simulink model "px42LoopCtr20210902"  (R2022a)
settings: Solver=FixedStepDiscrete  StartTime=0.0  StopTime=inf  FixedStep=0.005  RelTol=1e-3  EnableMultiTasking=on
InitFcn:
  | I_x = 0.00478;
  | I_y = 0.00502;
  | I_z = 0.00736;
  | m=1;
  | L=0.11667;
undefined symbols (not defined in the file): dev, DiscIntNeverNeededParam, Main, pwm_output0
libraries: simulink x30, px4lib x3, px4uORBlib x2, sharedtransform x1
(part 1 of 3)
settings Model: SimulationMode=external  ExtModeTrigDuration=10  Creator=The MathWorks, Inc.  LastModifiedBy=001
settings SolverCC: AlgebraicLoopSolver=TrustRegion  PositivePriorityOrder=on  AutoInsertRateTranBlk=on
settings DataIOCC: LimitDataPoints=on  MaxDataPoints=10000
settings OptimizationCC: BlockReduction=off  EnhancedBackFolding=on  PassReuseOutputArgsAs=Individual arguments  MaxStackSize=64  OptimizeBlockOrder=speed  DifferentSizesBufferReuse=on  OptimizationCustomize=off  EfficientTunableParamExpr=on
settings DebuggingCC: MultiTaskDSMMsg=none  ParameterTunabilityLossMsg=error  UnconnectedInputMsg=warning  UnconnectedOutputMsg=warning  UnconnectedLineMsg=warning  SFMachineParentedDataDiag=warning  ArithmeticOperatorsInVariantConditions=warning
settings HardwareCC: ProdBitPerPointer=32  ProdBitPerSizeT=32  ProdBitPerPtrDiffT=32  ProdLargestAtomicInteger=Long  ProdLargestAtomicFloat=Double  ProdWordSize=32  ProdLongLongMode=on  ProdHWDeviceType=ARM Compatible->ARM Cortex
settings SFSimCC: SimTargetLang=C++
settings RTWCC: SystemTargetFile=ert.tlc  HardwareBoard=PX4 Pixhawk 1  TLCOptions="-aInlineSetEventsForThisBaseRateFcn=TLC_FALSE -aSuppressMultiTaskScheduler=TLC_FALSE  -aRateBasedStepFcn=0"  TemplateMakefile=ert_default_tmf  GenerateReport=on  Toolchain=GNU Tools for PX4 Autopilots  IncludeHyperlinkInReport=on  LaunchReport=on  TargetLang=C++  GenerateTraceInfo=on  GenerateTraceReport=on  GenerateTraceReportSl=on  GenerateTraceReportSf=on  GenerateTraceReportEml=on
settings CodeAppCC: ForceParamTrailComments=on  IgnoreCustomStorageClasses=off  OperatorAnnotations=on  SimulinkDataObjDesc=on  SFDataObjDesc=on  InsertBlockDesc=on
settings ERTTargetCC: SupportNonInlinedSFcns=on  SupportVariableSizeSignals=on  ExtMode=on  ExtModeMexArgs='127.0.0.1' 1 17725

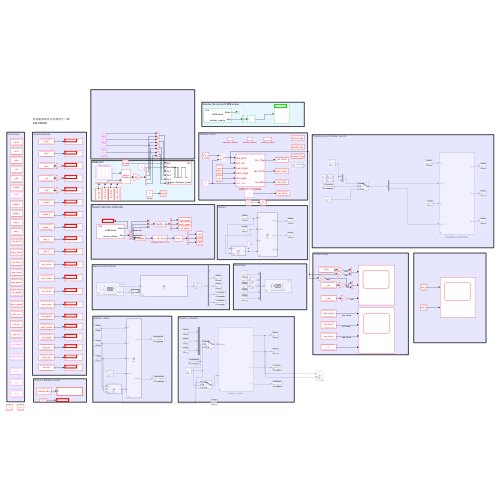
[thumbnail: Simulink's stored preview of the top-level diagram]
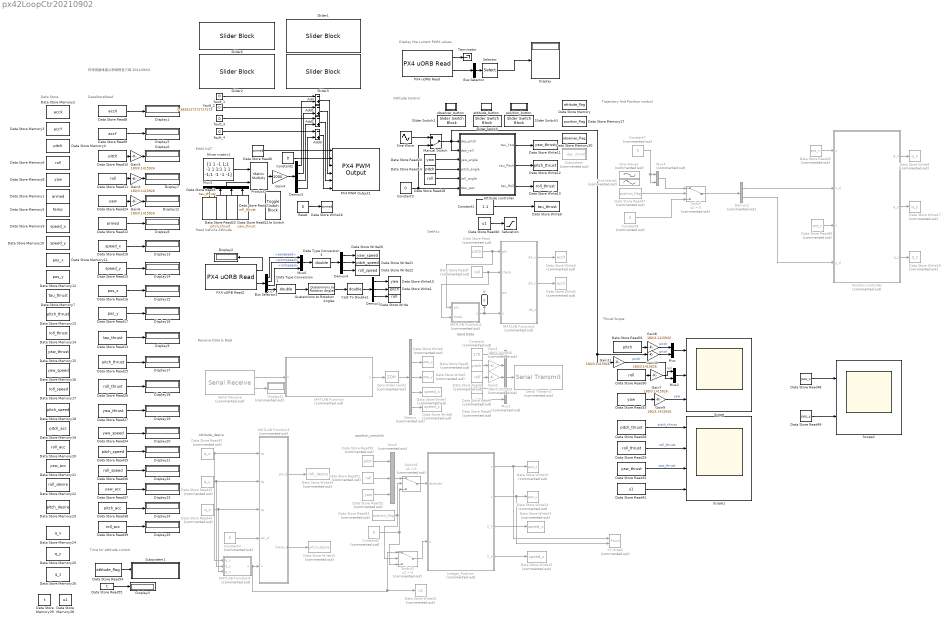
== system px42LoopCtr20210902 ==
  note: 将观测器维度从思维降至三维
      | 2021/09/02
  note: Time for attitude control
  note: position_simulink
  note: Trajectory And Position control
  note: Attitude_desire
  note: Thrust Scope
  note: Attitude Control
  note: DataStoreRead
  note: Receive Data & Deal
  note: Send Data
  note: Data Store
  note: Display the current PWM values
  note: PWM OUT
  note: Read Vehicle Attitude
  note: GetAcc
  Add{,1..3} (4 alike) : Sum  Inputs=-+  OutDataTypeStr=uint16
  Attitude controller : Subsystem
  Bus Selector : BusSelector  OutputSignals=output  OutputAsBus=on
  Bus Selector2 : BusSelector  OutputSignals=yawspeed,pitchspeed,rollspeed,q
  Cast To Double1 : DataTypeConversion  OutDataTypeStr=double  SaturateOnIntegerOverflow=off  RndMeth=Floor
  Constant : Constant  Commented=on  Value=170  OutDataTypeStr=double
  Constant1 : Constant  Value=1.1
  Constant2 : Constant  Value=0  OutDataTypeStr=boolean
  Constant3 : Constant  Value=0
  Constant4 : Constant  Commented=on  Value=0
  Constant5 : Constant  Commented=on  Value=0
  Constant7 : Constant  Commented=on  Value=5
  Constant8 : Constant  Commented=on  Value=0
  Data Store Memory : DataStoreMemory  DataStoreName=attitude_flag  ReadBeforeWriteMsg=warning  WriteAfterWriteMsg=warning  WriteAfterReadMsg=warning  ShowAdditionalParam=off  OutDataTypeStr=boolean
  Data Store Memory1 : DataStoreMemory  DataStoreName=armed  ReadBeforeWriteMsg=warning  WriteAfterWriteMsg=warning  WriteAfterReadMsg=warning  ShowAdditionalParam=off  OutDataTypeStr=boolean
  Data Store Memory10 : DataStoreMemory  DataStoreName=speed_y  ReadBeforeWriteMsg=warning  WriteAfterWriteMsg=warning  WriteAfterReadMsg=warning  ShowAdditionalParam=off  OutDataTypeStr=double
  Data Store Memory11 : DataStoreMemory  DataStoreName=pos_x  ReadBeforeWriteMsg=warning  WriteAfterWriteMsg=warning  WriteAfterReadMsg=warning  ShowAdditionalParam=off  OutDataTypeStr=double
  Data Store Memory12 : DataStoreMemory  DataStoreName=pos_y  ReadBeforeWriteMsg=warning  WriteAfterWriteMsg=warning  WriteAfterReadMsg=warning  ShowAdditionalParam=off  OutDataTypeStr=double
  Data Store Memory13 : DataStoreMemory  DataStoreName=pitch_thrust  ReadBeforeWriteMsg=warning  WriteAfterWriteMsg=warning  WriteAfterReadMsg=warning  ShowAdditionalParam=off  OutDataTypeStr=double
  Data Store Memory14 : DataStoreMemory  DataStoreName=roll_thrust  ReadBeforeWriteMsg=warning  WriteAfterWriteMsg=warning  WriteAfterReadMsg=warning  ShowAdditionalParam=off  OutDataTypeStr=double
  Data Store Memory15 : DataStoreMemory  DataStoreName=yaw_thrust  ReadBeforeWriteMsg=warning  WriteAfterWriteMsg=warning  WriteAfterReadMsg=warning  ShowAdditionalParam=off  OutDataTypeStr=double
  Data Store Memory16 : DataStoreMemory  DataStoreName=yaw_speed  ReadBeforeWriteMsg=warning  WriteAfterWriteMsg=warning  WriteAfterReadMsg=warning  ShowAdditionalParam=off  OutDataTypeStr=double
  Data Store Memory17 : DataStoreMemory  DataStoreName=roll_speed  ReadBeforeWriteMsg=warning  WriteAfterWriteMsg=warning  WriteAfterReadMsg=warning  ShowAdditionalParam=off  OutDataTypeStr=double
  Data Store Memory18 : DataStoreMemory  DataStoreName=pitch_speed  ReadBeforeWriteMsg=warning  WriteAfterWriteMsg=warning  WriteAfterReadMsg=warning  ShowAdditionalParam=off  OutDataTypeStr=double
  Data Store Memory19 : DataStoreMemory  DataStoreName=pitch_acc  ReadBeforeWriteMsg=warning  WriteAfterWriteMsg=warning  WriteAfterReadMsg=warning  ShowAdditionalParam=off  OutDataTypeStr=double
  Data Store Memory2 : DataStoreMemory  DataStoreName=accX  ReadBeforeWriteMsg=warning  WriteAfterWriteMsg=warning  WriteAfterReadMsg=warning  ShowAdditionalParam=off  OutDataTypeStr=double
  Data Store Memory20 : DataStoreMemory  DataStoreName=roll_acc  ReadBeforeWriteMsg=warning  WriteAfterWriteMsg=warning  WriteAfterReadMsg=warning  ShowAdditionalParam=off  OutDataTypeStr=double
  Data Store Memory21 : DataStoreMemory  DataStoreName=yaw_acc  ReadBeforeWriteMsg=warning  WriteAfterWriteMsg=warning  WriteAfterReadMsg=warning  ShowAdditionalParam=off  OutDataTypeStr=double
  Data Store Memory22 : DataStoreMemory  DataStoreName=roll_desire  ReadBeforeWriteMsg=warning  WriteAfterWriteMsg=warning  WriteAfterReadMsg=warning  ShowAdditionalParam=off  OutDataTypeStr=double
  Data Store Memory23 : DataStoreMemory  DataStoreName=pitch_desire  ReadBeforeWriteMsg=warning  WriteAfterWriteMsg=warning  WriteAfterReadMsg=warning  ShowAdditionalParam=off  OutDataTypeStr=double
  Data Store Memory24 : DataStoreMemory  DataStoreName=q_x  ReadBeforeWriteMsg=warning  WriteAfterWriteMsg=warning  WriteAfterReadMsg=warning  ShowAdditionalParam=off  OutDataTypeStr=double
  Data Store Memory25 : DataStoreMemory  DataStoreName=q_y  ReadBeforeWriteMsg=warning  WriteAfterWriteMsg=warning  WriteAfterReadMsg=warning  ShowAdditionalParam=off  OutDataTypeStr=double
  Data Store Memory26 : DataStoreMemory  DataStoreName=q_z  ReadBeforeWriteMsg=warning  WriteAfterWriteMsg=warning  WriteAfterReadMsg=warning  ShowAdditionalParam=off  OutDataTypeStr=double
  Data Store Memory27 : DataStoreMemory  DataStoreName=position_flag  ReadBeforeWriteMsg=warning  WriteAfterWriteMsg=warning  WriteAfterReadMsg=warning  ShowAdditionalParam=off  OutDataTypeStr=boolean
  Data Store Memory28 : DataStoreMemory  DataStoreName=u1  ReadBeforeWriteMsg=warning  WriteAfterWriteMsg=warning  WriteAfterReadMsg=warning  ShowAdditionalParam=off
  Data Store Memory29 : DataStoreMemory  DataStoreName=t  ReadBeforeWriteMsg=warning  WriteAfterWriteMsg=warning  WriteAfterReadMsg=warning  ShowAdditionalParam=off
  Data Store Memory3 : DataStoreMemory  DataStoreName=accY  ReadBeforeWriteMsg=warning  WriteAfterWriteMsg=warning  WriteAfterReadMsg=warning  ShowAdditionalParam=off  OutDataTypeStr=double
  Data Store Memory30 : DataStoreMemory  DataStoreName=observer_flag  ReadBeforeWriteMsg=warning  WriteAfterWriteMsg=warning  WriteAfterReadMsg=warning  ShowAdditionalParam=off  OutDataTypeStr=boolean
  Data Store Memory4 : DataStoreMemory  DataStoreName=pitch  ReadBeforeWriteMsg=warning  WriteAfterWriteMsg=warning  WriteAfterReadMsg=warning  ShowAdditionalParam=off  OutDataTypeStr=double
  Data Store Memory5 : DataStoreMemory  DataStoreName=temp  ReadBeforeWriteMsg=warning  WriteAfterWriteMsg=warning  WriteAfterReadMsg=warning  ShowAdditionalParam=off  OutDataTypeStr=double  Dimensions=5
  Data Store Memory6 : DataStoreMemory  DataStoreName=roll  ReadBeforeWriteMsg=warning  WriteAfterWriteMsg=warning  WriteAfterReadMsg=warning  ShowAdditionalParam=off  OutDataTypeStr=double
  Data Store Memory7 : DataStoreMemory  DataStoreName=tau_thrust  ReadBeforeWriteMsg=warning  WriteAfterWriteMsg=warning  WriteAfterReadMsg=warning  ShowAdditionalParam=off  OutDataTypeStr=double
  Data Store Memory8 : DataStoreMemory  DataStoreName=yaw  ReadBeforeWriteMsg=warning  WriteAfterWriteMsg=warning  WriteAfterReadMsg=warning  ShowAdditionalParam=off  OutDataTypeStr=double
  Data Store Memory9 : DataStoreMemory  DataStoreName=speed_x  ReadBeforeWriteMsg=warning  WriteAfterWriteMsg=warning  WriteAfterReadMsg=warning  ShowAdditionalParam=off  OutDataTypeStr=double
  Data Store Read : DataStoreRead  Commented=on  DataStoreName=pitch  IndexOptions=Index vector (dialog)  Indices=1  OutputSizes=1
  Data Store Read1 : DataStoreRead  Commented=on  DataStoreName=pitch  IndexOptions=Index vector (dialog)  Indices=1  OutputSizes=1
  Data Store Read10 : DataStoreRead  DataStoreName=pitch  IndexOptions=Index vector (dialog)  Indices=1  OutputSizes=1
  Data Store Read11 : DataStoreRead  DataStoreName=roll  IndexOptions=Index vector (dialog)  Indices=1  OutputSizes=1
  Data Store Read12 : DataStoreRead  DataStoreName=armed  IndexOptions=Index vector (dialog)  Indices=1  OutputSizes=1
  Data Store Read13 : DataStoreRead  DataStoreName=tau_thrust  IndexOptions=Index vector (dialog)  Indices=1  OutputSizes=1
  Data Store Read14 : DataStoreRead  DataStoreName=pitch  IndexOptions=Index vector (dialog)  Indices=1  OutputSizes=1
  Data Store Read15 : DataStoreRead  DataStoreName=speed_y  IndexOptions=Index vector (dialog)  Indices=1  OutputSizes=1
  Data Store Read16 : DataStoreRead  DataStoreName=pos_x  IndexOptions=Index vector (dialog)  Indices=1  OutputSizes=1
  Data Store Read17 : DataStoreRead  DataStoreName=pos_y  IndexOptions=Index vector (dialog)  Indices=1  OutputSizes=1
  Data Store Read18 : DataStoreRead  DataStoreName=roll  IndexOptions=Index vector (dialog)  Indices=1  OutputSizes=1
  Data Store Read19 : DataStoreRead  DataStoreName=speed_x  IndexOptions=Index vector (dialog)  Indices=1  OutputSizes=1
  Data Store Read2 : DataStoreRead  Commented=on  DataStoreName=roll  IndexOptions=Index vector (dialog)  Indices=1  OutputSizes=1
  Data Store Read20 : DataStoreRead  DataStoreName=yaw  IndexOptions=Index vector (dialog)  Indices=1  OutputSizes=1
  Data Store Read21 : DataStoreRead  DataStoreName=roll_thrust  IndexOptions=Index vector (dialog)  Indices=1  OutputSizes=1
  Data Store Read22 : DataStoreRead  DataStoreName=yaw_thrust  IndexOptions=Index vector (dialog)  Indices=1  OutputSizes=1
  Data Store Read23 : DataStoreRead  DataStoreName=pitch_thrust  IndexOptions=Index vector (dialog)  Indices=1  OutputSizes=1
  Data Store Read24 : DataStoreRead  DataStoreName=yaw  IndexOptions=Index vector (dialog)  Indices=1  OutputSizes=1
  Data Store Read25 : DataStoreRead  DataStoreName=pitch_thrust  IndexOptions=Index vector (dialog)  Indices=1  OutputSizes=1
  Data Store Read26 : DataStoreRead  DataStoreName=roll_thrust  IndexOptions=Index vector (dialog)  Indices=1  OutputSizes=1
  Data Store Read27 : DataStoreRead  DataStoreName=yaw_thrust  IndexOptions=Index vector (dialog)  Indices=1  OutputSizes=1
  Data Store Read28 : DataStoreRead  DataStoreName=pitch_thrust  IndexOptions=Index vector (dialog)  Indices=1  OutputSizes=1
  Data Store Read29 : DataStoreRead  DataStoreName=roll_thrust  IndexOptions=Index vector (dialog)  Indices=1  OutputSizes=1
  Data Store Read3 : DataStoreRead  DataStoreName=tau_thrust  IndexOptions=Index vector (dialog)  Indices=1  OutputSizes=1
  Data Store Read30 : DataStoreRead  DataStoreName=roll  IndexOptions=Index vector (dialog)  Indices=1  OutputSizes=1
  Data Store Read31 : DataStoreRead  DataStoreName=pitch  IndexOptions=Index vector (dialog)  Indices=1  OutputSizes=1
  Data Store Read32 : DataStoreRead  DataStoreName=yaw_thrust  IndexOptions=Index vector (dialog)  Indices=1  OutputSizes=1
  Data Store Read33 : DataStoreRead  DataStoreName=yaw  IndexOptions=Index vector (dialog)  Indices=1  OutputSizes=1
  Data Store Read34 : DataStoreRead  DataStoreName=yaw_speed  IndexOptions=Index vector (dialog)  Indices=1  OutputSizes=1
  Data Store Read35 : DataStoreRead  DataStoreName=pitch_speed  IndexOptions=Index vector (dialog)  Indices=1  OutputSizes=1
  Data Store Read36 : DataStoreRead  DataStoreName=roll_speed  IndexOptions=Index vector (dialog)  Indices=1  OutputSizes=1
  Data Store Read37 : DataStoreRead  DataStoreName=yaw_acc  IndexOptions=Index vector (dialog)  Indices=1  OutputSizes=1
  Data Store Read38 : DataStoreRead  DataStoreName=pitch_acc  IndexOptions=Index vector (dialog)  Indices=1  OutputSizes=1
  Data Store Read39 : DataStoreRead  DataStoreName=roll_acc  IndexOptions=Index vector (dialog)  Indices=1  OutputSizes=1
  Data Store Read4 : DataStoreRead  Commented=on  DataStoreName=accX  IndexOptions=Index vector (dialog)  Indices=1  OutputSizes=1
  Data Store Read40 : DataStoreRead  DataStoreName=u1  IndexOptions=Index vector (dialog)  Indices=1  OutputSizes=1
  Data Store Read41 : DataStoreRead  DataStoreName=u1  IndexOptions=Index vector (dialog)  Indices=1  OutputSizes=1
  Data Store Read42 : DataStoreRead  Commented=on  DataStoreName=q_x  IndexOptions=Index vector (dialog)  Indices=1  OutputSizes=1
  Data Store Read43 : DataStoreRead  Commented=on  DataStoreName=q_y  IndexOptions=Index vector (dialog)  Indices=1  OutputSizes=1
  Data Store Read44 : DataStoreRead  Commented=on  DataStoreName=q_z  IndexOptions=Index vector (dialog)  Indices=1  OutputSizes=1
  Data Store Read45 : DataStoreRead  Commented=on  DataStoreName=pos_x  IndexOptions=Index vector (dialog)  Indices=1  OutputSizes=1
  Data Store Read46 : DataStoreRead  Commented=on  DataStoreName=pos_y  IndexOptions=Index vector (dialog)  Indices=1  OutputSizes=1
  Data Store Read47 : DataStoreRead  Commented=on  DataStoreName=position_flag  IndexOptions=Index vector (dialog)  Indices=1  OutputSizes=1
  Data Store Read48 : DataStoreRead  DataStoreName=pos_x  IndexOptions=Index vector (dialog)  Indices=1  OutputSizes=1
  Data Store Read49 : DataStoreRead  DataStoreName=pos_y  IndexOptions=Index vector (dialog)  Indices=1  OutputSizes=1
  Data Store Read5 : DataStoreRead  Commented=on  DataStoreName=accY  IndexOptions=Index vector (dialog)  Indices=1  OutputSizes=1
  Data Store Read50 : DataStoreRead  Commented=on  DataStoreName=pitch  IndexOptions=Index vector (dialog)  Indices=1  OutputSizes=1
  Data Store Read51 : DataStoreRead  Commented=on  DataStoreName=roll  IndexOptions=Index vector (dialog)  Indices=1  OutputSizes=1
  Data Store Read52 : DataStoreRead  Commented=on  DataStoreName=yaw  IndexOptions=Index vector (dialog)  Indices=1  OutputSizes=1
  Data Store Read53 : DataStoreRead  Commented=on  DataStoreName=position_flag  IndexOptions=Index vector (dialog)  Indices=1  OutputSizes=1
  Data Store Read54 : DataStoreRead  DataStoreName=attitude_flag  IndexOptions=Index vector (dialog)  Indices=1  OutputSizes=1
  Data Store Read55 : DataStoreRead  DataStoreName=t  IndexOptions=Index vector (dialog)  Indices=1  OutputSizes=1
  Data Store Read6 : DataStoreRead  DataStoreName=armed  IndexOptions=Index vector (dialog)  Indices=1  OutputSizes=1
  Data Store Read7 : DataStoreRead  Commented=on  DataStoreName=roll  IndexOptions=Index vector (dialog)  Indices=1  OutputSizes=1
  Data Store Read8 : DataStoreRead  DataStoreName=accX  IndexOptions=Index vector (dialog)  Indices=1  OutputSizes=1
  Data Store Read9 : DataStoreRead  DataStoreName=accY  IndexOptions=Index vector (dialog)  Indices=1  OutputSizes=1
  Data Store Write : DataStoreWrite  DataStoreName=roll  IndexOptions=Index vector (dialog)  Indices=1  OutputSizes=1
  Data Store Write1 : DataStoreWrite  DataStoreName=pitch  IndexOptions=Index vector (dialog)  Indices=1  OutputSizes=1
  Data Store Write10 : DataStoreWrite  DataStoreName=yaw  IndexOptions=Index vector (dialog)  Indices=1  OutputSizes=1
  Data Store Write11 : DataStoreWrite  DataStoreName=yaw_thrust  IndexOptions=Index vector (dialog)  Indices=1  OutputSizes=1
  Data Store Write12 : DataStoreWrite  DataStoreName=pitch_thrust  IndexOptions=Index vector (dialog)  Indices=1  OutputSizes=1
  Data Store Write13 : DataStoreWrite  DataStoreName=roll_thrust  IndexOptions=Index vector (dialog)  Indices=1  OutputSizes=1
  Data Store Write14 : DataStoreWrite  Commented=on  DataStoreName=roll_desire  IndexOptions=Index vector (dialog)  Indices=1  OutputSizes=1
  Data Store Write15 : DataStoreWrite  Commented=on  DataStoreName=pitch_desire  IndexOptions=Index vector (dialog)  Indices=1  OutputSizes=1
  Data Store Write16 : DataStoreWrite  DataStoreName=armed  IndexOptions=Index vector (dialog)  Indices=1  OutputSizes=1
  Data Store Write17 : DataStoreWrite  Commented=on  DataStoreName=q_y  IndexOptions=Index vector (dialog)  Indices=1  OutputSizes=1
  Data Store Write18 : DataStoreWrite  Commented=on  DataStoreName=q_z  IndexOptions=Index vector (dialog)  Indices=1  OutputSizes=1
  Data Store Write19 : DataStoreWrite  Commented=on  DataStoreName=pos_x  IndexOptions=Index vector (dialog)  Indices=1  OutputSizes=1
  Data Store Write2 : DataStoreWrite  Commented=on  DataStoreName=accY  IndexOptions=Index vector (dialog)  Indices=1  OutputSizes=1
  Data Store Write20 : DataStoreWrite  DataStoreName=yaw_speed  IndexOptions=Index vector (dialog)  Indices=1  OutputSizes=1
  Data Store Write21 : DataStoreWrite  DataStoreName=pitch_speed  IndexOptions=Index vector (dialog)  Indices=1  OutputSizes=1
  Data Store Write22 : DataStoreWrite  DataStoreName=roll_speed  IndexOptions=Index vector (dialog)  Indices=1  OutputSizes=1
  Data Store Write23 : DataStoreWrite  Commented=on  DataStoreName=pos_y  IndexOptions=Index vector (dialog)  Indices=1  OutputSizes=1
  Data Store Write24 : DataStoreWrite  Commented=on  DataStoreName=speed_x  IndexOptions=Index vector (dialog)  Indices=1  OutputSizes=1
  Data Store Write25 : DataStoreWrite  Commented=on  DataStoreName=speed_x  IndexOptions=Index vector (dialog)  Indices=1  OutputSizes=1
  Data Store Write26 : DataStoreWrite  Commented=on  DataStoreName=u1  IndexOptions=Index vector (dialog)  Indices=1  OutputSizes=1
  Data Store Write3 : DataStoreWrite  Commented=on  DataStoreName=accX  IndexOptions=Index vector (dialog)  Indices=1  OutputSizes=1
  Data Store Write4 : DataStoreWrite  Commented=on  DataStoreName=q_x  IndexOptions=Index vector (dialog)  Indices=1  OutputSizes=1
  Data Store Write5 : DataStoreWrite  Commented=on  DataStoreName=pos_y  IndexOptions=Index vector (dialog)  Indices=1  OutputSizes=1
  Data Store Write6 : DataStoreWrite  Commented=on  DataStoreName=pos_x  IndexOptions=Index vector (dialog)  Indices=1  OutputSizes=1
  Data Store Write7 : DataStoreWrite  Commented=on  DataStoreName=speed_x  IndexOptions=Index vector (dialog)  Indices=1  OutputSizes=1
  Data Store Write8 : DataStoreWrite  Commented=on  DataStoreName=speed_y  IndexOptions=Index vector (dialog)  Indices=1  OutputSizes=1
  Data Store Write9 : DataStoreWrite  DataStoreName=tau_thrust  IndexOptions=Index vector (dialog)  Indices=1  OutputSizes=1
  Data Type Conversion1 : DataTypeConversion  OutDataTypeStr=double  SaturateOnIntegerOverflow=off  RndMeth=Floor
  Data Type Conversion3 : DataTypeConversion  OutDataTypeStr=double  SaturateOnIntegerOverflow=off  RndMeth=Floor
  Demux : Demux  Commented=on  Outputs=5
  Demux1 : Demux  Outputs=3
  Demux2 : Demux  Commented=on  Outputs=2
  Demux3 : Demux
  Demux4 : Demux  Outputs=3
  Display{,1..3,5..9,12..25} (23 alike) : Display
  Display11 : Display  Commented=on
  Gain1 : Gain  Commented=on  Gain=180/3.1415926
  Gain{3,5..11} (8 alike) : Gain  Gain=180/3.1415926
  Gain2 : Gain  Commented=on  Gain=180/3.1415926
  Gain4 : Gain  Gain=1000  OutDataTypeStr=uint16
  Integer_Position : Subsystem  Commented=on
  MATLAB Function : MATLAB Function  Commented=on  TreatAsAtomicUnit=on
  MATLAB Function1 : MATLAB Function  Commented=on  TreatAsAtomicUnit=on
  MATLAB Function2 : MATLAB Function  Commented=on  TreatAsAtomicUnit=on
  MATLAB Function3 : MATLAB Function  Commented=on  TreatAsAtomicUnit=on
  MATLAB Function4 : MATLAB Function  Commented=on  TreatAsAtomicUnit=on
  Manual Switch : ManualSwitch  CurrentSetting=0
  Mixer matrix1 : Constant  Value=[1 1 -1 1;1 -1 1 1;1 1 1 -1;1 -1 -1 -1]  OutDataTypeStr=Inherit: Inherit via back propagation
  Mux : Mux  Inputs=2
  Mux1 : Mux  Commented=on  Inputs=5
  Mux2 : Mux  Inputs=2
  Mux3 : Mux
  Mux4 : Mux  Commented=on  Inputs=2
  Mux5 : Mux  Commented=on  Inputs=3
  Mux6 : Mux  Inputs=3
  PX4 PWM Output1 : px4lib/PX4 PWM Output  pwmDevice=Main (/dev/pwm_output0)  pwmChannel1_=on  pwmChannel2_=on  pwmChannel3_=on  pwmChannel4_=on  pwmChannel5_=off  pwmChannel6_=off  pwmChannel7_=off  pwmChannel8_=off  forceTerminateFailsafe=off  outputErrorStatus=off
      settings: SourceProductBaseCode=PX4AUTOPILOTS
  PX4 uORB Read : px4uORBlib/PX4 uORB Read  uORBTopic=actuator_outputs  selectInstance=actuator_outputs  SampleTime=0.01  BlockingMode=off  BlockTimeout=1e-3
      settings: SourceProductBaseCode=PX4AUTOPILOTS
  PX4 uORB Read2 : px4uORBlib/PX4 uORB Read  uORBTopic=vehicle_attitude  selectInstance=vehicle_attitude  SampleTime=0.005  BlockingMode=off  BlockTimeout=1e-3
      settings: SourceProductBaseCode=PX4AUTOPILOTS
  Position controller : Subsystem  Commented=on
  Product2 : Product  Multiplication=Matrix(*)  RndMeth=Zero
  Quaternions to Rotation Angles : sharedtransform/Quaternions to Rotation Angles  rotationOrder=ZYX  aMode=aMode
      settings: SourceProductBaseCode=AE,PW,DR,MT,VE
  Reset : Constant  Value=0  OutDataTypeStr=boolean  SampleTime=-1
      settings: OpenFcn=|
      | if strcmp('0',get_param(gcb, 'Value'))                        set_param(gcb, 'Value', '1');
      | else
      |             set_param(gcb, 'Value', '0');
      | end
  Saturation : Saturate  UpperLimit=1.2  LowerLimit=1
  Scope : Scope  NumInputPorts=3
  Scope1 : Scope  NumInputPorts=4
  Scope2 : Scope  NumInputPorts=2
  Selector : Selector  InputPortWidth=16  IndexOptions=Select all  Indices=[1 4]  OutputSizes=1
  Serial Receive : px4lib/Serial Receive  Commented=on  SCIModule=/dev/ttyS6  DataType=uint8  DataLength=96  OutputStatus=on  SampleTime=0.1  BlockingMode=on  PartialData=on  Timeout=5
      settings: SourceProductBaseCode=PX4AUTOPILOTS
  Serial Transmit : px4lib/Serial Transmit  Commented=on  SCIModule=/dev/ttyS6
      settings: SourceProductBaseCode=PX4AUTOPILOTS
  Sine Wave : Sin  Amplitude=pi/18  Frequency=pi/5
  Sine Wave1 : Sin  Commented=on  Amplitude=5  Bias=-5  Frequency=pi/20  Phase=pi/2
  Sine Wave2 : Sin  Commented=on  Amplitude=5  Frequency=pi/20
  Slider Switch : SliderSwitchBlock
      settings: Values={{'Off', 'On'}, [0 1]}
  Slider Switch1 : SliderSwitchBlock
      settings: Values={{'Off', 'On'}, [0 1]}
  Slider Switch2 : SliderSwitchBlock
      settings: Values={{'Off', 'On'}, [0 1]}
  Slider{1..3,6} (4 alike) : SliderBlock  ScaleMax=200
  Subsystem : Subsystem  Commented=on
  Subsystem1 : Subsystem
  Switch : Switch  Commented=on  Criteria=u2 > Threshold  SaturateOnIntegerOverflow=off  InputSameDT=off
  Switch1 : Switch  Commented=on  Criteria=u2 > Threshold  SaturateOnIntegerOverflow=off  InputSameDT=off
  Switch2 : Switch  Commented=on  Criteria=u2 > Threshold  SaturateOnIntegerOverflow=off  InputSameDT=off
  Terminator : Terminator
  Toggle Switch : ToggleSwitchBlock
      settings: Values={{'Off', 'On'}, [0 1]}
  XY Graph : Record  Commented=on  FileSettingsInternal="{\"entries\":[{\"content\":{\"excelSettings\":{\"content\":{},\"type\":\"Streamout.ExcelSettings\"}},\"type\":\"Streamout.FileSettingStorage\",\"uuid\":\"6213bd28-0707-420c-b9d0-85ec00109663\"}],\"packageUris\":[\"http://schema.mathworks.com/mf0/streamout_blocks/R2020a\"],\"version\":\"1.0\"}"  Layout=[1 1]  SignalsInternal="{\"entries\":[{\"content\":{\"signals\":[{\"content\":{\"blockPath\":[\"px42LoopCtr20210902/XY Graph\"],\"channel\":[],\"dimensions\":[1],\"domain\":\"px42LoopCtr20210902/XY Graph\",\"lineColor\":\"#a2142f\",\"plots\":[1],\"port\":1,\"sid\":[],\"signalID\":26,\"signalName\":\"XY Graph:1\"},\"type\":\"RecordBlkView.Signal\",\"uuid\":\"ca54dc8b-01c9-48b3-91c8-992ebf1b532a\"},{\"content\":{\"blockPath\":[\"px42LoopCtr20210902/XY Graph\"],\"channel\":[],\"dimensions\":[1],\"domain\":\"px42LoopCtr20210902/XY Graph\",\"lineColor\":\"#139fff\",\"plots\":[1],\"port\":2,\"sid\":[],\"signalID\":29,\"signalName\":\"XY Graph:2\"},\"type\":\"RecordBlkView.Signal\",\"uuid\":\"be6928dd-ca14-4b52-8b65-118c23c18760\"}]},\"type\":\"RecordBlkView.InputSignals\",\"uuid\":\"45dc4eb5-cd21-48fb-aeff-c90ae330fbe6\"}],\"packageUris\":[\"http://schema.mathworks.com/mf0/streamout_blocks/R2020a\"],\"version\":\"1.0\"}"  VisualizationBindings="{\"xyplotplugin\":{\"info\":[{\"series\":[{\"bindingParametersList\":[{\"parameter\":\"X-Axis\",\"signalID\":26,\"signalName\":\"XY Graph:1\"},{\"parameter\":\"Y-Axis\",\"signalID\":29,\"signalName\":\"XY Graph:2\"}],\"seriesID\":23335}],\"subplotID\":1}]}}"  CompatibilityTag=XY  st=-1
  Zero-Order Hold1 : ZeroOrderHold  Commented=on  SampleTime=-1
  attitude_button : Subsystem
  fault_1 : Constant  Value=0
  fault_2 : Constant  Value=0.3835227272727273
  fault_3 : Constant  Value=0
  fault_4 : Constant  Value=0
  observer_button : Subsystem
  position_button : Subsystem
  u : Outport
  wires:
  PX4 uORB Read/1 -> Terminator/1
  PX4 uORB Read/2 -> Bus Selector/1
  Bus Selector/1 -> Selector/1
  Selector/1 -> Display/1
  PX4 uORB Read2/1 -> Display2/1
  Quaternions to Rotation Angles/1 -> Cast To Double1/1
  Data Type Conversion1/1 -> Quaternions to Rotation Angles/1
  Bus Selector2/4 -> Data Type Conversion1/1  "<q>"
  PX4 uORB Read2/2 -> Bus Selector2/1
  Demux1/3 -> Data Store Write/1
  Demux1/2 -> Data Store Write1/1
  Mux1/1 -> Serial Transmit/1
  Data Store Read1/1 -> Gain1/1
  Data Store Read2/1 -> Gain2/1
  Cast To Double1/1 -> Demux1/1
  Gain1/1 -> Mux1/2
  Data Store Read4/1 -> Mux1/4
  Gain2/1 -> Mux1/3
  Data Store Read5/1 -> Mux1/5
  Constant/1 -> Mux1/1
  Demux/3 -> Data Store Write5/1
  Demux/4 -> Data Store Write7/1
  Demux/5 -> Data Store Write8/1
  MATLAB Function/1(y) -> Zero-Order Hold1/1
  Serial Receive/1 -> MATLAB Function/1(u)
  Serial Receive/2 -> Display11/1
  Zero-Order Hold1/1 -> Demux/1
  Demux/2 -> Data Store Write6/1
  MATLAB Function1/2(dd_y) -> Data Store Write2/1
  Data Store Read7/1 -> MATLAB Function1/2(theta), MATLAB Function2/2(theta)
  MATLAB Function2/1(u) -> u/1, MATLAB Function1/4(u)
  Data Store Read/1 -> MATLAB Function2/1(phi), MATLAB Function1/1(phi)
  MATLAB Function1/1(dd_x) -> Data Store Write3/1
  Data Store Read8/1 -> Display1/1
  Data Store Read9/1 -> Display5/1
  Data Store Read12/1 -> Display8/1
  Data Store Read19/1 -> Display13/1
  Data Store Read16/1 -> Display15/1
  Data Store Read17/1 -> Display16/1
  Data Store Read15/1 -> Display14/1
  Data Store Read13/1 -> Display9/1
  Mux3/1 -> Product2/2
  Product2/1 -> Gain4/1
  Gain4/1 -> Demux3/1
  Data Store Read3/1 -> Mux3/1
  Data Store Read6/1 -> PX4 PWM Output1/1
  Data Store Read11/1 -> Gain3/1
  Gain3/1 -> Display7/1
  Data Store Read10/1 -> Gain5/1
  Gain5/1 -> Display6/1
  Data Store Read14/1 -> Attitude controller/4(pitch_angle)
  Data Store Read18/1 -> Attitude controller/5("roll_angle ")
  Demux1/1 -> Data Store Write10/1
  Data Store Read20/1 -> Attitude controller/3(yaw_angle)
  Attitude controller/1(tau_Yaw) -> Data Store Write11/1
  Attitude controller/2(tau_Pitch) -> Data Store Write12/1
  Attitude controller/3(tau_Roll) -> Data Store Write13/1
  Data Store Read22/1 -> Mux3/4
  Data Store Read25/1 -> Display17/1
  Data Store Read26/1 -> Display18/1
  Data Store Read27/1 -> Display19/1
  Data Store Read28/1 -> Scope1/1  "pitch_thrust"
  Data Store Read24/1 -> Gain6/1
  Gain6/1 -> Display12/1
  Gain8/1 -> Mux/1  "pitch"
  Data Store Read31/1 -> Gain8/1
  Data Store Read30/1 -> Gain7/1
  Data Store Read29/1 -> Scope1/2  "roll_thrust"
  Data Store Read33/1 -> Gain9/1
  Gain9/1 -> Scope/3  "yaw"
  Data Store Read32/1 -> Scope1/3  "yaw_thrust"
  Data Store Read34/1 -> Display20/1
  Data Store Read35/1 -> Display21/1
  Data Store Read36/1 -> Display22/1
  Data Store Read38/1 -> Display24/1
  Data Store Read39/1 -> Display25/1
  Data Store Read37/1 -> Display23/1
  Bus Selector2/2 -> Mux6/2  "<pitchspeed>"
  Bus Selector2/3 -> Mux6/3  "<rollspeed>"
  Bus Selector2/1 -> Mux6/1  "<yawspeed>"
  Mux6/1 -> Data Type Conversion3/1
  Data Type Conversion3/1 -> Demux4/1
  Demux4/1 -> Data Store Write20/1
  Demux4/2 -> Data Store Write21/1
  Demux4/3 -> Data Store Write22/1
  Constant4/1 -> MATLAB Function3/4(psi_d)
  MATLAB Function4/1(u) -> Switch2/1, Data Store Write26/1, MATLAB Function3/5(u)
  Data Store Read43/1 -> MATLAB Function4/2(q_y), MATLAB Function3/2(qy)
  Data Store Read42/1 -> MATLAB Function4/1(q_x), MATLAB Function3/1(qx)
  MATLAB Function3/1(phi_d) -> Data Store Write14/1
  MATLAB Function3/2(theta_d) -> Data Store Write15/1
  Reset/1 -> Data Store Write16/1
  Constant2/1 -> PX4 PWM Output1/2
  Data Store Read44/1 -> MATLAB Function4/3(q_z), MATLAB Function3/3(qz)
  Position controller/1(q_x) -> Data Store Write4/1
  Position controller/2(q_y) -> Data Store Write17/1
  Position controller/3(q_z) -> Data Store Write18/1
  Data Store Read45/1 -> Position controller/1(x)
  Data Store Read46/1 -> Position controller/3(y)
  Mixer matrix1/1 -> Product2/1
  Mux/1 -> Scope/1
  Mux2/1 -> Scope/2
  Gain7/1 -> Mux2/1  "roll"
  Mux4/1 -> Switch/1
  Constant8/1 -> Switch/3
  Data Store Read47/1 -> Switch/2
  Switch/1 -> Demux2/1
  Demux2/1 -> Position controller/2(x_d)
  Demux2/2 -> Position controller/4(y_d)
  Data Store Read48/1 -> Scope2/1
  Data Store Read49/1 -> Scope2/2
  Data Store Read50/1 -> Mux5/1
  Data Store Read51/1 -> Mux5/2
  Data Store Read52/1 -> Mux5/3
  Integer_Position/1(x) -> XY Graph/1, Data Store Write19/1
  Integer_Position/2(y) -> XY Graph/2, Data Store Write23/1
  Integer_Position/3(V_Y) -> Data Store Write24/1
  Integer_Position/4(V_X) -> Data Store Write25/1
  Switch1/1 -> Integer_Position/1(Attitude)
  Mux5/1 -> Switch1/1
  Data Store Read53/1 -> Switch2/2, Switch1/2
  Constant5/1 -> Switch2/3, Switch1/3
  Switch2/1 -> Integer_Position/2(u)
  Constant3/1 -> Manual Switch/2, Attitude controller/6(des_yaw)
  Constant7/1 -> Mux4/2, Mux4/1
  Data Store Read41/1 -> Scope1/4
  Data Store Read40/1 -> Saturation/1
  Constant1/1 -> Data Store Write9/1
  Data Store Read54/1 -> Subsystem1/Enable
  Data Store Read55/1 -> Display3/1
  Data Store Read23/1 -> Mux3/2
  Data Store Read21/1 -> Mux3/3
  fault_1/1 -> Add/1
  fault_2/1 -> Add1/1
  fault_3/1 -> Add2/1
  fault_4/1 -> Add3/1
  Demux3/1 -> Add/2
  Demux3/2 -> Add1/2
  Demux3/3 -> Add2/2
  Demux3/4 -> Add3/2
  Add/1 -> PX4 PWM Output1/3
  Add1/1 -> PX4 PWM Output1/4
  Add2/1 -> PX4 PWM Output1/5
  Add3/1 -> PX4 PWM Output1/6
  Sine Wave/1 -> Manual Switch/1
  Manual Switch/1 -> Gain11/1, Gain10/1, Attitude controller/2(des_roll), Attitude controller/1(des_pitch)
  Gain10/1 -> Mux/2  "pitch"
  Gain11/1 -> Mux2/2  "pitch"

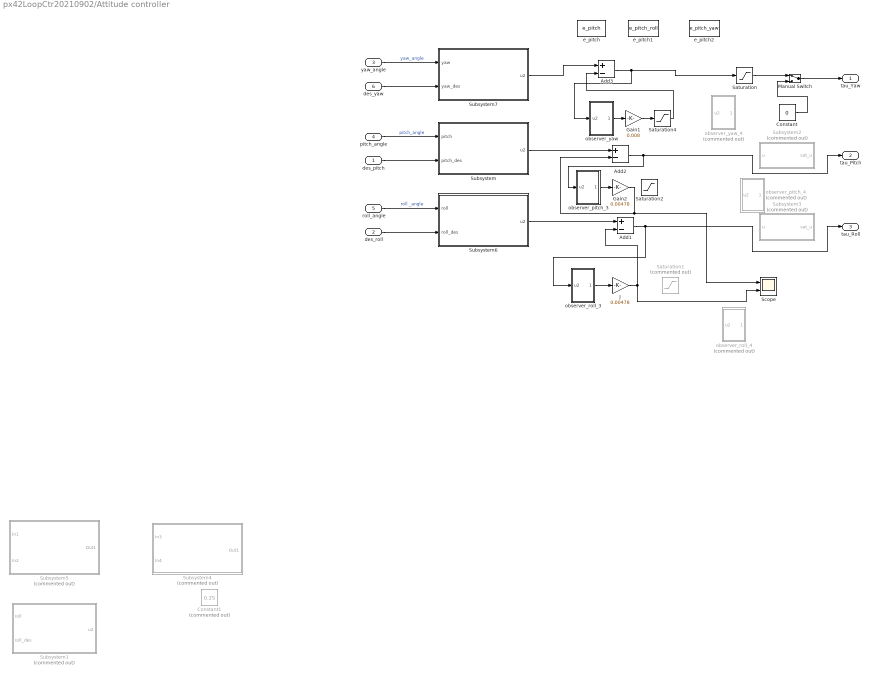
== system px42LoopCtr20210902/Attitude controller ==
  des_pitch : Inport
  des_roll : Inport  Port=2
  yaw_angle : Inport  Port=3
  pitch_angle : Inport  Port=4
  "roll_angle " : Inport  Port=5
  des_yaw : Inport  Port=6
  Add1 : Sum  Inputs=+-
  Add2 : Sum  Inputs=+-
  Add3 : Sum  Inputs=+-
  Constant : Constant  Value=0
  Constant1 : Constant  Commented=on  Value=0.25
  Gain1 : Gain  Gain=0.008
  Gain2 : Gain  Gain=0.00478
  J : Gain  Gain=0.00478
  Manual Switch : ManualSwitch
  Saturation : Saturate  UpperLimit=0.1  LowerLimit=-0.1
  Saturation1 : Saturate  Commented=on  UpperLimit=0.2
  Saturation2 : Saturate  UpperLimit=0.2
  Saturation4 : Saturate  UpperLimit=0.2
  Scope : Scope  NumInputPorts=2
  Subsystem : Subsystem
  Subsystem1 : Subsystem  Commented=on
  Subsystem2 : Subsystem  Commented=on
  Subsystem3 : Subsystem  Commented=on
  Subsystem4 : Subsystem  Commented=on  mask{c=1, g=1}
      mask prompts: c "gain_1"; g "gain_2"
  Subsystem5 : Subsystem  Commented=on  mask{c=1, g=1}
      mask prompts: c "gain_1"; g "gain_2"
  Subsystem6 : Subsystem
  Subsystem7 : Subsystem
  e_pitch : DataStoreMemory  DataStoreName=e_pitch  ReadBeforeWriteMsg=warning  WriteAfterWriteMsg=warning  WriteAfterReadMsg=warning  ShowAdditionalParam=off
  e_pitch1 : DataStoreMemory  DataStoreName=e_pitch_roll  ReadBeforeWriteMsg=warning  WriteAfterWriteMsg=warning  WriteAfterReadMsg=warning  ShowAdditionalParam=off
  e_pitch2 : DataStoreMemory  DataStoreName=e_pitch_yaw  ReadBeforeWriteMsg=warning  WriteAfterWriteMsg=warning  WriteAfterReadMsg=warning  ShowAdditionalParam=off
  observer_pitch_3 : Subsystem
  observer_pitch_4 : Subsystem  Commented=on
  observer_roll_3 : Subsystem
  observer_roll_4 : Subsystem  Commented=on
  observer_yaw : Subsystem
  observer_yaw_4 : Subsystem  Commented=on
  tau_Yaw : Outport
  tau_Pitch : Outport  Port=2
  tau_Roll : Outport  Port=3
  wires:
  Saturation/1 -> Manual Switch/1
  Constant/1 -> Manual Switch/2
  Subsystem/1(u2) -> Add2/1
  Add2/1 -> observer_pitch_3/1(u2), tau_Pitch/1
  des_pitch/1 -> Subsystem/2(pitch_des)
  pitch_angle/1 -> Subsystem/1(pitch)  "pitch_angle"
  Manual Switch/1 -> tau_Yaw/1
  "roll_angle "/1 -> Subsystem6/1(roll)  "roll _angle"
  des_roll/1 -> Subsystem6/2(roll_des)
  yaw_angle/1 -> Subsystem7/1(yaw)  "yaw_angle"
  des_yaw/1 -> Subsystem7/2(yaw_des)
  Add1/1 -> observer_roll_3/1(u2), tau_Roll/1
  Subsystem6/1(u2) -> Add1/1
  Saturation4/1 -> Add3/2
  Gain1/1 -> Saturation4/1
  Add3/1 -> observer_yaw/1(u2), Saturation/1
  Subsystem7/1(u2) -> Add3/1
  observer_yaw/1(Out1) -> Gain1/1
  observer_roll_3/1(Out1) -> J/1
  observer_pitch_3/1(Out1) -> Gain2/1
  J/1 -> Scope/2, Add1/2
  Gain2/1 -> Scope/1, Add2/2

== system px42LoopCtr20210902/Integer_Position ==
  Attitude : Inport
  u : Inport  Port=2
  Demux : Demux  Outputs=3
  Demux2 : Demux  Outputs=3
  Intgrt_dX : DiscreteIntegrator  gainval=1  SampleTime=-1  ICPrevOutput=DiscIntNeverNeededParam  ICPrevScaledInput=DiscIntNeverNeededParam
  Intgrt_dY : DiscreteIntegrator  gainval=1  SampleTime=-1  ICPrevOutput=DiscIntNeverNeededParam  ICPrevScaledInput=DiscIntNeverNeededParam
  Intgrt_dZ : DiscreteIntegrator  gainval=1  SampleTime=-1  LowerSaturationLimit=0  ICPrevOutput=DiscIntNeverNeededParam  ICPrevScaledInput=DiscIntNeverNeededParam
  Intgrt_ddX : DiscreteIntegrator  gainval=1  SampleTime=-1  ICPrevOutput=DiscIntNeverNeededParam  ICPrevScaledInput=DiscIntNeverNeededParam
  Intgrt_ddY : DiscreteIntegrator  gainval=1  SampleTime=-1  ICPrevOutput=DiscIntNeverNeededParam  ICPrevScaledInput=DiscIntNeverNeededParam
  Intgrt_ddZ : DiscreteIntegrator  gainval=1  SampleTime=-1  ICPrevOutput=DiscIntNeverNeededParam  ICPrevScaledInput=DiscIntNeverNeededParam
  MATLAB Function1 : MATLAB Function  TreatAsAtomicUnit=on
  Mux2 : Mux  Inputs=3
  Saturation : Saturate  UpperLimit=inf  LowerLimit=0
  slower3 : Gain
  slower4 : Gain
  slower5 : Gain
  x : Outport
  y : Outport  Port=2
  V_Y : Outport  Port=3
  V_X : Outport  Port=4
  wires:
  Saturation/1 -> Mux2/3
  Intgrt_ddY/1 -> V_Y/1, Intgrt_dY/1
  Intgrt_ddX/1 -> Intgrt_dX/1, V_X/1
  Intgrt_dX/1 -> Mux2/1
  Mux2/1 -> Demux2/1
  Attitude/1 -> Demux/1
  Demux/3 -> MATLAB Function1/3(psi)
  Demux/2 -> MATLAB Function1/2(theta)
  Intgrt_dY/1 -> Mux2/2
  Demux/1 -> MATLAB Function1/1(phi)
  slower3/1 -> Intgrt_ddX/1
  Intgrt_dZ/1 -> Saturation/1
  Intgrt_ddZ/1 -> Intgrt_dZ/1
  MATLAB Function1/1(dd_x) -> slower3/1
  MATLAB Function1/2(dd_y) -> slower4/1
  slower4/1 -> Intgrt_ddY/1
  slower5/1 -> Intgrt_ddZ/1
  MATLAB Function1/3(dd_z) -> slower5/1
  Demux2/1 -> x/1
  Demux2/2 -> y/1
  u/1 -> MATLAB Function1/4(u)

== system px42LoopCtr20210902/Position controller ==
  x : Inport
  x_d : Inport  Port=2
  y : Inport  Port=3
  y_d : Inport  Port=4
  Constant : Constant  Value=0
  Gain2 : Gain  Gain=0.1
  Gain4 : Gain  Gain=0.1
  Saturation1 : Saturate
  Saturation2 : Saturate
  Subsystem1 : Subsystem  mask{c=1, g=1}
      mask prompts: c "gain_1"; g "gain_2"
  Subsystem3 : Subsystem  mask{c=1, g=1}
      mask prompts: c "gain_1"; g "gain_2"
  q_x : Outport
  q_y : Outport  Port=2
  q_z : Outport  Port=3
  wires:
  Constant/1 -> q_z/1
  y_d/1 -> Subsystem1/2(In2)  "y_d"
  y/1 -> Subsystem1/1(In1)  "y"
  Gain2/1 -> Saturation1/1
  Saturation1/1 -> q_y/1
  Subsystem1/1(Out1) -> Gain2/1
  Saturation2/1 -> q_x/1
  Gain4/1 -> Saturation2/1
  Subsystem3/1(Out1) -> Gain4/1
  x_d/1 -> Subsystem3/2(In2)  "x_d"
  x/1 -> Subsystem3/1(In1)  "x"

== system px42LoopCtr20210902/Subsystem ==
  Constant7 : Constant  Value=0
  Data Store Read54 : DataStoreRead  DataStoreName=position_flag  IndexOptions=Index vector (dialog)  Indices=1  OutputSizes=1
  Data Store Read55 : DataStoreRead  DataStoreName=pitch_desire  IndexOptions=Index vector (dialog)  Indices=1  OutputSizes=1
  Data Store Read56 : DataStoreRead  DataStoreName=roll_desire  IndexOptions=Index vector (dialog)  Indices=1  OutputSizes=1
  Mux7 : Mux  Inputs=2
  Switch3 : Switch  Criteria=u2 > Threshold  SaturateOnIntegerOverflow=off  InputSameDT=off
  des_pitch/roll : Outport
  wires:
  Switch3/1 -> des_pitch/roll/1
  Mux7/1 -> Switch3/1
  Constant7/1 -> Switch3/3
  Data Store Read55/1 -> Mux7/1
  Data Store Read54/1 -> Switch3/2
  Data Store Read56/1 -> Mux7/2

== system px42LoopCtr20210902/Subsystem1 ==
  Enable : EnablePort
  Constant9 : Constant
  Data Store Write27 : DataStoreWrite  DataStoreName=t  IndexOptions=Index vector (dialog)  Indices=1  OutputSizes=1
  Discrete-Time Integrator : DiscreteIntegrator  SampleTime=-1  ICPrevOutput=DiscIntNeverNeededParam  ICPrevScaledInput=DiscIntNeverNeededParam
  wires:
  Constant9/1 -> Discrete-Time Integrator/1
  Discrete-Time Integrator/1 -> Data Store Write27/1

== system px42LoopCtr20210902/attitude_button ==
  Data Store Write28 : DataStoreWrite  DataStoreName=attitude_flag  IndexOptions=Index vector (dialog)  Indices=1  OutputSizes=1
  attitude_flag : Constant  Value=0  OutDataTypeStr=boolean
  wires:
  attitude_flag/1 -> Data Store Write28/1

== system px42LoopCtr20210902/observer_button ==
  Data Store Write28 : DataStoreWrite  DataStoreName=observer_flag  IndexOptions=Index vector (dialog)  Indices=1  OutputSizes=1
  observer_flag : Constant  Value=0  OutDataTypeStr=boolean
  wires:
  observer_flag/1 -> Data Store Write28/1

== system px42LoopCtr20210902/position_button ==
  Data Store Write28 : DataStoreWrite  DataStoreName=position_flag  IndexOptions=Index vector (dialog)  Indices=1  OutputSizes=1
  position_flag : Constant  Value=0  OutDataTypeStr=boolean
  wires:
  position_flag/1 -> Data Store Write28/1

== system px42LoopCtr20210902/Attitude controller/Subsystem ==
  pitch : Inport
  pitch_des : Inport  Port=2
  Add : Sum  Inputs=+----
  Add1 : Sum  Inputs=+-
  Add2 : Sum  Inputs=+-
  Constant1 : Constant  Value=0
  Data Store Read : DataStoreRead  DataStoreName=attitude_flag  IndexOptions=Index vector (dialog)  Indices=1  OutputSizes=1
  Data Store Read1 : DataStoreRead  DataStoreName=pitch_speed  IndexOptions=Index vector (dialog)  Indices=1  OutputSizes=1
  Data Store Write : DataStoreWrite  DataStoreName=e_pitch  IndexOptions=Index vector (dialog)  Indices=1  OutputSizes=1
  Demux : Demux  Outputs=3
  Discrete Derivative1 : simulink/Discrete/Discrete Derivative  gainval=1.0  ICPrevScaledInput=0.0  OutMin=[]  OutMax=[]  OutDataType=fixdt(1, 16)  OutScaling=2^-10  DoSatur=off
  Gain : Gain  Gain=0.01/0.0052
  Gain1 : Gain  Gain=0.00502
  Mux : Mux  Inputs=3
  Product : Product  Inputs=3
  Product1 : Product
  Sign : Signum
  Slider : SliderBlock  ScaleMax=20
  Slider1 : SliderBlock  ScaleMax=20
  Slider2 : SliderBlock  ScaleMin=2  ScaleMax=10
  Slider3 : SliderBlock  ScaleMax=20
  Slider4 : SliderBlock  ScaleMax=10
  Subsystem1 : Subsystem
  Switch : Switch  Criteria=u2 > Threshold  SaturateOnIntegerOverflow=off  InputSameDT=off
  b : Constant  Value=2.470900809716599
  l : Constant  Value=0.5282118055555556
  u2 : Outport
  wires:
  Product/1 -> Add/3
  Add1/1 -> Sign/1, Product/1  "v-v*"
  Demux/3 -> Gain/1, Add1/1  "v"
  pitch/1 -> Mux/1
  Discrete Derivative1/1 -> Add/1  "v*_dot"
  l/1 -> Product1/2
  b/1 -> Subsystem1/3(b), Product/3
  Subsystem1/2(H) -> Product/2
  Subsystem1/1(v*) -> Add1/2, Discrete Derivative1/1
  Sign/1 -> Product1/1
  Add/1 -> Gain1/1
  pitch_des/1 -> Mux/2
  Add2/1 -> Data Store Write/1, Add/2
  Product1/1 -> Add/4
  Gain/1 -> Add/5
  Gain1/1 -> u2/1
  Data Store Read/1 -> Switch/2
  Switch/1 -> Demux/1
  Constant1/1 -> Switch/3
  Mux/1 -> Switch/1
  Demux/1 -> Subsystem1/1(pitch), Add2/1
  Demux/2 -> Subsystem1/2(pitch_des), Add2/2
  Data Store Read1/1 -> Mux/3

== system px42LoopCtr20210902/Attitude controller/Subsystem1 ==
  roll : Inport
  roll_des : Inport  Port=2
  Add : Sum  Inputs=+----
  Add1 : Sum  Inputs=+-
  Add2 : Sum  Inputs=+-
  Discrete Derivative : simulink/Discrete/Discrete Derivative  gainval=1.0  ICPrevScaledInput=0.0  OutMin=[]  OutMax=[]  OutDataType=fixdt(1, 16)  OutScaling=2^-10  DoSatur=off
  Discrete Derivative1 : simulink/Discrete/Discrete Derivative  gainval=1.0  ICPrevScaledInput=0.0  OutMin=[]  OutMax=[]  OutDataType=fixdt(1, 16)  OutScaling=2^-10  DoSatur=off
  Gain : Gain  Gain=0.01/0.00478
  Gain1 : Gain  Gain=0.00478
  Product : Product  Inputs=3
  Product1 : Product
  Sign : Signum
  Subsystem1 : Subsystem
  b : Constant
  l : Constant  Value=0
  u2 : Outport
  wires:
  Product/1 -> Add/3
  Add1/1 -> Sign/1, Product/1  "v-v*"
  Discrete Derivative/1 -> Gain/1, Add1/1  "v"
  roll/1 -> Discrete Derivative/1, Subsystem1/1(roll), Add2/1
  Discrete Derivative1/1 -> Add/1  "v*_dot"
  l/1 -> Product1/2
  b/1 -> Subsystem1/3(b), Product/3
  Subsystem1/2(H) -> Product/2
  Subsystem1/1(v*) -> Add1/2, Discrete Derivative1/1
  Sign/1 -> Product1/1
  Add/1 -> Gain1/1
  roll_des/1 -> Subsystem1/2(roll_des), Add2/2
  Add2/1 -> Add/2
  Product1/1 -> Add/4
  Gain/1 -> Add/5
  Gain1/1 -> u2/1

== system px42LoopCtr20210902/Attitude controller/Subsystem2 ==
  u : Inport
  Add : Sum
  Add1 : Sum  Inputs=+-
  Add2 : Sum
  Divide : Product  Inputs=*/
  Gain : Gain  Gain=0.5
  Gain1 : Gain  Gain=0.5
  Gain2 : Gain  Gain=sqrt(pi)/2
  MATLAB Function : MATLAB Function  TreatAsAtomicUnit=on
  Product : Product
  Product2 : Product
  Sign : Signum
  lower bound : Constant  Value=0.5
  upper bound : Constant  Value=0.5
  sat_u : Outport
  wires:
  Add2/1 -> Product2/1, Divide/2  "tm"
  lower bound/1 -> Add1/2, Add/2
  u/1 -> Sign/1, Gain2/1
  Sign/1 -> Product/2
  Add1/1 -> Gain1/1
  Product/1 -> Add2/2
  upper bound/1 -> Add/1, Add1/1
  Gain1/1 -> Product/1
  Gain2/1 -> Divide/1
  Gain/1 -> Add2/1
  Add/1 -> Gain/1
  Divide/1 -> MATLAB Function/1(u)
  MATLAB Function/1(y) -> Product2/2
  Product2/1 -> sat_u/1

== system px42LoopCtr20210902/Attitude controller/Subsystem3 ==
  u : Inport
  Add : Sum
  Add1 : Sum  Inputs=+-
  Add2 : Sum
  Divide : Product  Inputs=*/
  Gain : Gain  Gain=0.5
  Gain1 : Gain  Gain=0.5
  Gain2 : Gain  Gain=sqrt(pi)/2
  MATLAB Function : MATLAB Function  TreatAsAtomicUnit=on
  Product : Product
  Product2 : Product
  Sign : Signum
  lower bound : Constant  Value=0.4
  upper bound : Constant  Value=0.4
  sat_u : Outport
  wires:
  Product2/1 -> sat_u/1
  MATLAB Function/1(y) -> Product2/2
  Divide/1 -> MATLAB Function/1(u)
  Add/1 -> Gain/1
  Gain/1 -> Add2/1
  Gain2/1 -> Divide/1
  Gain1/1 -> Product/1
  upper bound/1 -> Add1/1, Add/1
  Product/1 -> Add2/2
  Add1/1 -> Gain1/1
  Sign/1 -> Product/2
  u/1 -> Gain2/1, Sign/1
  lower bound/1 -> Add/2, Add1/2
  Add2/1 -> Divide/2, Product2/1  "tm"

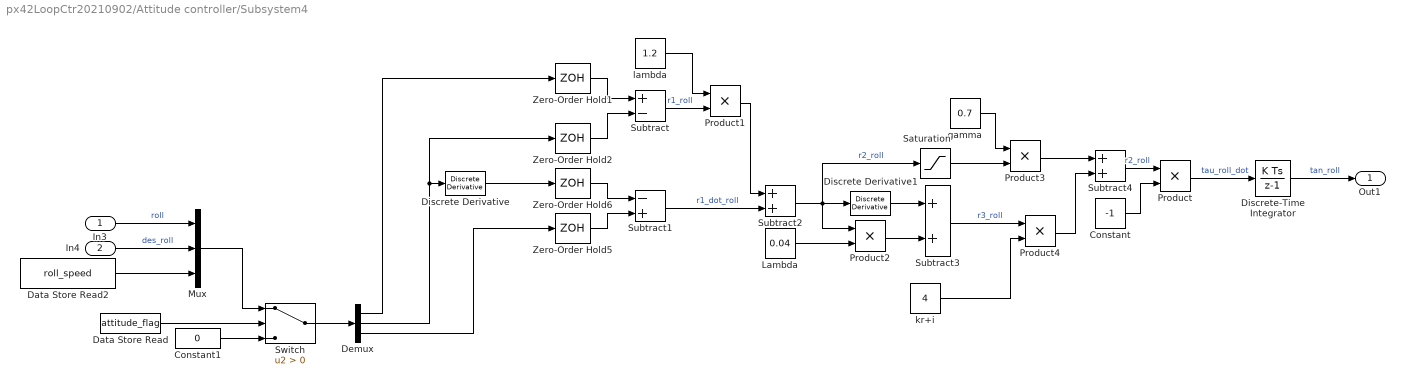
== system px42LoopCtr20210902/Attitude controller/Subsystem4 ==
  In3 : Inport
  In4 : Inport  Port=2
  Constant : Constant  Value=-1
  Constant1 : Constant  Value=0
  Data Store Read : DataStoreRead  DataStoreName=attitude_flag  IndexOptions=Index vector (dialog)  Indices=1  OutputSizes=1
  Data Store Read2 : DataStoreRead  DataStoreName=roll_speed  IndexOptions=Index vector (dialog)  Indices=1  OutputSizes=1
  Demux : Demux  Outputs=3
  Discrete Derivative : simulink/Discrete/Discrete Derivative  gainval=1.0  ICPrevScaledInput=0.0  OutMin=[]  OutMax=[]  OutDataType=fixdt(1, 16)  OutScaling=2^-10  DoSatur=off
  Discrete Derivative1 : simulink/Discrete/Discrete Derivative  gainval=1.0  ICPrevScaledInput=0.0  OutMin=[]  OutMax=[]  OutDataType=fixdt(1, 16)  OutScaling=2^-10  DoSatur=off
  Discrete-Time Integrator : DiscreteIntegrator  SampleTime=-1  ICPrevOutput=DiscIntNeverNeededParam  ICPrevScaledInput=DiscIntNeverNeededParam
  Lambda : Constant  Value=0.04
  Mux : Mux  Inputs=3
  Product{,1..4} (5 alike) : Product
  Saturation : Saturate  UpperLimit=1  LowerLimit=-1
  Subtract : Sum  Inputs=+-
  Subtract1 : Sum  Inputs=-+
  Subtract2 : Sum
  Subtract3 : Sum
  Subtract4 : Sum
  Switch : Switch  Criteria=u2 > Threshold  SaturateOnIntegerOverflow=off  InputSameDT=off
  Zero-Order Hold{1..2,5..6} (4 alike) : ZeroOrderHold  SampleTime=-1
  gamma : Constant  Value=0.7
  kr+i : Constant  Value=4
  lambda : Constant  Value=1.2
  Out1 : Outport
  wires:
  In3/1 -> Mux/1  "roll"
  In4/1 -> Mux/2  "des_roll"
  Zero-Order Hold1/1 -> Subtract/1
  Zero-Order Hold2/1 -> Subtract/2
  Subtract/1 -> Product1/2  "r1_roll"
  Data Store Read2/1 -> Mux/3
  Discrete Derivative/1 -> Zero-Order Hold6/1
  Zero-Order Hold5/1 -> Subtract1/2
  Zero-Order Hold6/1 -> Subtract1/1
  Subtract1/1 -> Subtract2/2  "r1_dot_roll"
  Product1/1 -> Subtract2/1
  Subtract2/1 -> Product2/1, Saturation/1, Discrete Derivative1/1  "r2_roll"
  Discrete Derivative1/1 -> Subtract3/1
  Product2/1 -> Subtract3/2
  Subtract3/1 -> Product4/1  "r3_roll"
  Saturation/1 -> Product3/2
  Product3/1 -> Subtract4/1
  Product4/1 -> Subtract4/2
  Subtract4/1 -> Product/1  "r2_roll"
  Constant/1 -> Product/2
  Product/1 -> Discrete-Time Integrator/1  "tau_roll_dot"
  Discrete-Time Integrator/1 -> Out1/1  "tan_roll"
  Constant1/1 -> Switch/3
  Data Store Read/1 -> Switch/2
  Mux/1 -> Switch/1
  Switch/1 -> Demux/1
  Demux/1 -> Zero-Order Hold1/1
  Demux/2 -> Zero-Order Hold2/1, Discrete Derivative/1
  Demux/3 -> Zero-Order Hold5/1
  lambda/1 -> Product1/1
  Lambda/1 -> Product2/2
  gamma/1 -> Product3/1
  kr+i/1 -> Product4/2

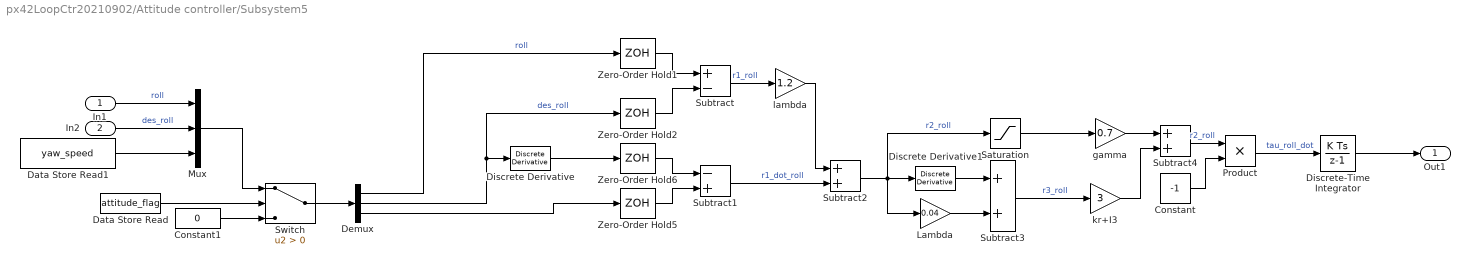
== system px42LoopCtr20210902/Attitude controller/Subsystem5 ==
  In1 : Inport
  In2 : Inport  Port=2
  Constant : Constant  Value=-1
  Constant1 : Constant  Value=0
  Data Store Read : DataStoreRead  DataStoreName=attitude_flag  IndexOptions=Index vector (dialog)  Indices=1  OutputSizes=1
  Data Store Read1 : DataStoreRead  DataStoreName=yaw_speed  IndexOptions=Index vector (dialog)  Indices=1  OutputSizes=1
  Demux : Demux  Outputs=3
  Discrete Derivative : simulink/Discrete/Discrete Derivative  gainval=1.0  ICPrevScaledInput=0.0  OutMin=[]  OutMax=[]  OutDataType=fixdt(1, 16)  OutScaling=2^-10  DoSatur=off
  Discrete Derivative1 : simulink/Discrete/Discrete Derivative  gainval=1.0  ICPrevScaledInput=0.0  OutMin=[]  OutMax=[]  OutDataType=fixdt(1, 16)  OutScaling=2^-10  DoSatur=off
  Discrete-Time Integrator : DiscreteIntegrator  SampleTime=-1  ICPrevOutput=DiscIntNeverNeededParam  ICPrevScaledInput=DiscIntNeverNeededParam
  Lambda : Gain  Gain=0.04
  Mux : Mux  Inputs=3
  Product : Product
  Saturation : Saturate  UpperLimit=1  LowerLimit=-1
  Subtract : Sum  Inputs=+-
  Subtract1 : Sum  Inputs=-+
  Subtract2 : Sum
  Subtract3 : Sum
  Subtract4 : Sum
  Switch : Switch  Criteria=u2 > Threshold  SaturateOnIntegerOverflow=off  InputSameDT=off
  Zero-Order Hold{1..2,5..6} (4 alike) : ZeroOrderHold  SampleTime=-1
  gamma : Gain  Gain=0.7
  kr+I3 : Gain  Gain=3
  lambda : Gain  Gain=1.2
  Out1 : Outport
  wires:
  Subtract3/1 -> kr+I3/1  "r3_roll"
  gamma/1 -> Subtract4/1
  Subtract2/1 -> Saturation/1, Lambda/1, Discrete Derivative1/1  "r2_roll"
  Subtract4/1 -> Product/1  "r2_roll"
  Discrete Derivative1/1 -> Subtract3/1
  kr+I3/1 -> Subtract4/2
  lambda/1 -> Subtract2/1
  Zero-Order Hold2/1 -> Subtract/2
  Constant/1 -> Product/2
  Saturation/1 -> gamma/1
  Lambda/1 -> Subtract3/2
  Discrete Derivative/1 -> Zero-Order Hold6/1
  Zero-Order Hold5/1 -> Subtract1/2
  Zero-Order Hold1/1 -> Subtract/1
  Demux/3 -> Zero-Order Hold5/1
  Subtract1/1 -> Subtract2/2  "r1_dot_roll"
  Zero-Order Hold6/1 -> Subtract1/1
  Subtract/1 -> lambda/1  "r1_roll"
  Demux/2 -> Zero-Order Hold2/1, Discrete Derivative/1  "des_roll"
  Product/1 -> Discrete-Time Integrator/1  "tau_roll_dot"
  Demux/1 -> Zero-Order Hold1/1  "roll"
  Switch/1 -> Demux/1
  Data Store Read/1 -> Switch/2
  Mux/1 -> Switch/1
  In1/1 -> Mux/1  "roll"
  In2/1 -> Mux/2  "des_roll"
  Data Store Read1/1 -> Mux/3
  Constant1/1 -> Switch/3
  Discrete-Time Integrator/1 -> Out1/1
